simulink model "LegoBalance_no_loop"  (Simulink 7.8)
settings: Solver=ode45  StartTime=0.0  StopTime=Tend  FixedStep=0.01  RelTol=1e-3
values from neighbouring files (symbols this model uses):
  A = zeros(2)    [analysis.m]
  B = A(:,1)    [analysis.m]
  C = [1 0]    [analysis.m]
  D = 0    [analysis.m]
  den0 = Dob    [analysis.m]
  den0_num0 = den0 + num0    [analysis.m]
  den1 = Dob    [analysis.m]
  initial = [theta_IC thetaDot_IC]'    [analysis.m]
  num1 = [C_fn(4) C_fn(3)]    [analysis.m]
  Tsamp = 0.001    [analysis.m]
settings Model: Creator=Robert  LastModifiedBy=ghost
settings SolverCC: AlgebraicLoopSolver=LineSearch
settings DataIOCC: SignalLoggingSaveFormat=Dataset
settings GRTTargetCC: CombineOutputUpdateFcns=on

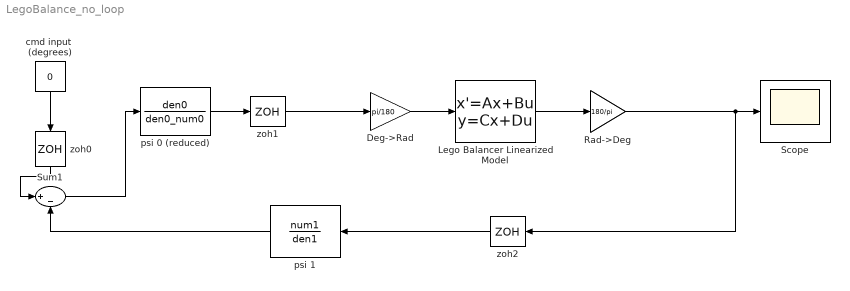
== system LegoBalance_no_loop ==
  Deg->Rad : Gain  Gain=pi/180
  Lego Balancer Linearized Model : StateSpace  A=A  B=B  C=C  D=D  X0=initial  ContinuousStateAttributes='theta'
  Rad->Deg : Gain  Gain=180/pi
  Scope : Scope
      settings: TimeRange=10  YMin=-1  YMax=3
  Sum1 : Sum  Inputs=|+-  SampleTime=Tsamp
  "cmd input  (degrees) " : Constant  Value=0
  psi 0 (reduced) : DiscreteTransferFcn  Numerator=den0  Denominator=den0_num0  SampleTime=Tsamp
  psi 1 : DiscreteTransferFcn  Numerator=num1  Denominator=den1  SampleTime=Tsamp
  zoh0 : ZeroOrderHold  SampleTime=Tsamp
  zoh1 : ZeroOrderHold  SampleTime=Tsamp
  zoh2 : ZeroOrderHold  SampleTime=Tsamp
  wires:
  zoh2/1 -> psi 1/1
  Sum1/1 -> psi 0 (reduced)/1
  psi 0 (reduced)/1 -> zoh1/1
  Lego Balancer Linearized Model/1 -> Rad->Deg/1
  zoh1/1 -> Deg->Rad/1
  Rad->Deg/1 -> zoh2/1, Scope/1
  Deg->Rad/1 -> Lego Balancer Linearized Model/1
  psi 1/1 -> Sum1/2
  "cmd input  (degrees) "/1 -> zoh0/1
  zoh0/1 -> Sum1/1
